simulink model "flightControlSystem"  (R2021a)
settings: Solver=ode3  StartTime=0  StopTime=TFinal  FixedStep=Ts  RelTol=1e-3  EnableMultiTasking=on
undefined symbols (not defined in the file): BINARIZATION_THRESHOLD, CHANGE_DERIVATIVE_ERROR_THRESHOLD_CURVE, CHANGE_DERIVATIVE_ERROR_THRESHOLD_STRAIGHT, codertarget, COG_X, COG_Y, Controller, DELAY_LANDING, DERIVATIVE_GAIN, DILATE_KERNEL, DiscIntNeverNeededParam, Discrete, DISK_KERNEL, Estimator, FLAG_WAIT_FOR_HOVERING, FOV, FRAME_SIZE_HEIGHT, FRAME_SIZE_WIDTH, g, G_B_GAIN, GAIN_LANDING, GAIN_TRACK, init, MAX_RADIUS_CROWN, MIN_RADIUS_CROWN, Sensors, strel, Time, TIME_HOLD, Ts, var_acc_angle_N, var_bias_gyr_N, var_gyro_p_N, Vehicle, Z_HIGH, Z_LOW
libraries: simulink x40, pid_lib x4, ctrlSharedLib x4, sharedtransform x3, visionmorphops x2, parrotlib x1
(part 3 of 3)

== matlab function flightControlSystem/Control System/Path Planning/MATLAB Function ==
  data: x_err_tr input; x_error output; y_err_tr input; x_err_ea input; y_err_ea input; flag_ho input; y_error output; flag_tl input
function [x_error, y_error] = decision_making(x_err_tr, y_err_tr, x_err_ea, ...
    y_err_ea, flag_ho, flag_tl)
% The MALTAB function sends the error along x- and y-axis to the non-linear 
% path planner. When the "flag_tl" is low, the position errors are computed
% as the difference between the end-marker and the drone CoG. Instead, when 
% the flag is high, the errors are computed by the difference between the 
% track and drone CoG.
%
% Inputs:
% - x_err_tr: tracking error along the x-axis. The error is expressed in 
% pixels.
% - y_err_tr: tracking error along the y-axis. The error is expressed in 
% pixels.
% - x_err_ea: position error along the x-axis when the end-marker is 
% detected. The error is expressed in pixels.
% - y_err_ea: position error along the y-axis when the end-marker is
% detected. The error is expressed in pixels.
% - flag_ho: the flag allows to check if the drone is able to fly.
% - flag_tl: the flag allows to trace the lane. 
%   
% Outputs
% - x_error: error between the drone CoG and the track/end-marker along the 
% x-axis. The error is expressed in pixels.
% - y_error: error between the drone CoG and the track/end-marker along the
% y-axis. The error is expressed in pixels

if flag_ho == 1
    
    if flag_tl == 0
        
        x_error = x_err_ea;
        y_error = y_err_ea;
        
    else
        
        x_error = x_err_tr;
        y_error = y_err_tr;

    end
    
else
    x_error = 0;
    y_error = 0;
    
end
    
end

== matlab function flightControlSystem/Image Processing System/track_VTP_generator ==
  data: frame input; error_y_track output; x_ref_prev input; y_ref_prev input; flag_track_prev input; error_x_track output; orientation_track output; flag_track output boolean; MIN_RADIUS_CROWN parameter; MAX_RADIUS_CROWN parameter; FOV parameter; COG_X parameter; COG_Y parameter
function [error_y_track, error_x_track, orientation_track, flag_track] = ...
track_VTP_generator(frame, x_ref_prev, y_ref_prev, flag_track_prev, ...
MIN_RADIUS_CROWN, MAX_RADIUS_CROWN, FOV, COG_X, COG_Y)
% The MATLAB function computes the error along x and y-axis between
% the drone COG (Center of Gravity) and the point of the track extract 
% by using of a crown circular mask. This errors is later used by the Path 
% Planner for the track tracking.  
%
%
% Inputs:
% - frame: binarized frame
% - x_ref_prev: previous value of the tracking point along the x-axis of 
% the track line. It is used as a reference for tracking the path.
% - y_ref_prev: previous value of the tracking point along the y-axis of 
% the track line. It is used as a reference for tracking the path.                                                                                                                                              
% - flag_track_prev: previous value assumed by the flag variablle, i.e., 
% the previous state of the drone (over the track / not over the track).
%
%
% Outputs:
% - error_y_track: error between the CoG of the drone and a point of the 
% lane in the forward direction along the y-axis. It is expressed in
% pixels.
% - error_x_track: error between the CoG of the drone and a point of the 
% lane in the forward direction along the x-axis. It is expressed in pixels. 
% - flag_track: it indicates if the drone is currently over the track (TRUE).
% - yaw: the heading angle of the track in the image plane.
%
%
% Parameters:
% - MIN_RADIUS_CROWN: minimum value of the radius of the crown mask. It is
% expressed in pixels.
% - MAX_RADIUS_CROWN: maximum value of the radius of the crown mask. It is
% expressed in pixels.
% - FOV: a portion of the crown used to detect the lane. It is expressed in
% radians.
% - COG_X: position of the drone CoG along x-axis of the reference frame.
% - COG_Y: position of the drone CoG along y-axis of the reference frame.

persistent x_accumulator
persistent y_accumulator
persistent pixel_count

if isempty(x_accumulator)
    x_accumulator = 0;
end

if isempty(y_accumulator)
    y_accumulator = 0;
end

if isempty(pixel_count)
    pixel_count = 0;
end

% the previous value of the heading angle of the lane 
orientation_track = atan2(-x_ref_prev,y_ref_prev); 
orientation_track = mod(orientation_track,2*pi);

% checking if the drone is over the lane
if flag_track_prev     

    % the set of pixels inside the crown mask
    for i = (COG_X-MAX_RADIUS_CROWN):(COG_X+MAX_RADIUS_CROWN) 

        for j = (COG_Y-MAX_RADIUS_CROWN):(COG_Y+MAX_RADIUS_CROWN)

            norm = sqrt(((i-(COG_X-0.5))^2)+((j-(COG_Y-0.5))^2));

            if norm >= MIN_RADIUS_CROWN && norm <= MAX_RADIUS_CROWN 

                axis_x = (i-(COG_X-0.5));
                axis_y = (j-(COG_Y-0.5));
                yaw_point_temp = atan2(axis_x,axis_y);


                yaw_point_temp_2 = mod(yaw_point_temp,2*pi);

                % a portion of the crown mask depending on the FOV
                threshold_1 = mod((orientation_track+(pi/FOV)),2*pi);

                threshold_2 = mod((orientation_track-(pi/FOV)),2*pi);

                if threshold_1 < threshold_2

                    flag_threshold = ...
                        (yaw_point_temp_2 <= 2*pi  && yaw_point_temp_2 >= threshold_2) ...
                        || (yaw_point_temp_2 <= threshold_1  && yaw_point_temp_2 >= 0);

                else

                    flag_threshold = ...
                        yaw_point_temp_2 <= threshold_1  && yaw_point_temp_2 >= threshold_2;

                end

                if flag_threshold
 
                    if frame(i,j)==1 
                        
                        pixel_count = pixel_count + 1;
                        x_accumulator = x_accumulator + i;
                        y_accumulator = y_accumulator + j;

                    end

                end

            end

        end
    end
    
else
    % checking for the initial heading angle of the lane. It can be 
    % different from the heading angle of the drone
    for i = (COG_X-MAX_RADIUS_CROWN):(COG_X+MAX_RADIUS_CROWN)

        for j = (COG_Y-MAX_RADIUS_CROWN):(COG_Y+MAX_RADIUS_CROWN)
            
            norm=sqrt(((i-(COG_X-0.5))^2)+((j-(COG_Y-0.5))^2));

            if norm>=MIN_RADIUS_CROWN && norm <= MAX_RADIUS_CROWN 

                 axis_x = (i-(COG_X-0.5));
                 axis_y = (j-(COG_Y-0.5));
                if frame(i,j)==1 
                    pixel_count=pixel_count +1;
                    x_accumulator=x_accumulator+i;
                    y_accumulator=y_accumulator+j;
                end
            end
        end
    end
end

% calculating the medium point of the lane as output of the mask
x_ref_temp = -(round(x_accumulator/pixel_count)-COG_X);
y_ref_temp = (round(y_accumulator/pixel_count)-COG_Y);

% when there is no track, the x_ref_temp and y_ref_temp variables are NaN.
% Below is the code for fix the issue.

if isnan(x_ref_temp)
    
    % if the computer vision algorithm does not detect the track, the 
    % drone position does not change
    error_x_track = 0 ;
    flag_error_x = false;
    
else
    
    % if the computer vision algorithm detects the track, a new position 
    % is computed for the tracking problem
    flag_error_x = true;
    error_x_track = x_ref_temp;
    
end

% As for the x coordinate
if isnan(y_ref_temp)
    
    error_y_track = 0 ;
    flag_error_y = false;
    
else
    
    error_y_track = y_ref_temp;
    flag_error_y=true ;
    
end

% checking if the drone is over the lane
flag_track = flag_error_x || flag_error_y;

% reset of the persistent variables
pixel_count = 0;
x_accumulator = 0;
y_accumulator = 0;

end

== stateflow chart flightControlSystem/Control System/Path Planning/circle count ==
  state State [group]
    - TAKE_OFF: The drone takes off and hovers.
    - LEAVE_MARKER: The drone leaves the marker through tracing the VTP set at the track.
    - TRACE_LANE: The drone traces either straight or curve line.
    - APPROACH_MARKER_CENTER: When the error between the drone CoG and the marker
    center is less than MAX_ERROR_LANDING, the drone flies down and then rises back.
  state INPUT [group]
    - flag_hover: flag raised when the drone is hovering within the altitude threshold.
    - flag_marker: flag raised when the marker is detected by the IPS.
  state OUTPUT [group]
    - cirlce_count: counting the circles that the drone has passed.
    - flag_tracelane: flag raised when the drone is going to track the lane.
  state TAKE_OFF
  state LEAVE_MARKER
    entry:
    flag_tracelane = 1;
  state TRACE_LANE
    entry:
    flag_tracelane = 1;
  state APPROACH_MARKER_CENTER
    entry:
    circle_count = circle_count +1
    flag_tracelane = 0
  (default) -> TAKE_OFF : {circle_count = 0, flag_tracelane = 0}
  TAKE_OFF -> LEAVE_MARKER : [after(3,sec) && flag_hover ==1]
  LEAVE_MARKER -> TRACE_LANE : [flag_hover == 1 && flag_end_marker == 0]
  APPROACH_MARKER_CENTER -> LEAVE_MARKER : [flag_hover == 0]
  TRACE_LANE -> APPROACH_MARKER_CENTER : [flag_end_marker == 1 ]
  data: flag_hover input; circle_count output; flag_end_marker input; flag_tracelane output

== matlab function flightControlSystem/Control System/Controller/Position Controller/Position error transformation (Earth to Body frame) ==
  data: yaw input; xy_err_earth input; xy_err_body output
function xy_err_body = fcn(yaw,xy_err_earth)

transformation = [cos(yaw), sin(yaw); -sin(yaw),  cos(yaw)];
xy_err_body = transformation * xy_err_earth;


end

== matlab function flightControlSystem/Control System/Path Planning/Non linear Path Planner/X_PLANNER/x_derivative_contribute /MATLAB Function ==
  data: derivative_error input; flag_change_error output; CHANGE_DERIVATIVE_ERROR_THRESHOLD input
function flag_change_error = change_error_checker(derivative_error, ...
    CHANGE_DERIVATIVE_ERROR_THRESHOLD)
% This MATLAB function recognizes if the derivative of the error is greater
% than a threshold value, i.e., the  CHANGE_DERIVATIVE_ERROR_THRESHOLD. 
% 
% Input:
% - derivative_error: derivative of the error. The error is expressed in 
% pixels
%
% Parameter:
% - CHANGE_DERIVATIVE_ERROR_THRESHOLD: threshold value.
%
% Output:
% - flag_change_error: flag raised when the derivative of the error
% changes.

if abs(derivative_error) >= CHANGE_DERIVATIVE_ERROR_THRESHOLD

    flag_change_error = 1;

else

    flag_change_error = 0;

end

== matlab function flightControlSystem/Control System/Path Planning/Non linear Path Planner/X_PLANNER/x_derivative_contribute /derivative error ==
  data: dev_contribute_prev input; derivative_error input; flag_change_error input; dev_contribute output; count_prev input; count output; flag_count_prev input; flag_count output; Ts parameter; TIME_HOLD parameter; DERIVATIVE_GAIN parameter
  function [dev_contribute, count, flag_count] = derivative_error(dev_contribute_prev, ...
    derivative_error, flag_change_error,count_prev,flag_count_prev, Ts, ...
    TIME_HOLD, DERIVATIVE_GAIN)
% This MATLAB function computes the derivative contribution of the path planner
% for the x coordinate.
%
% Inputs:
% - dev_contribute_prev: previous value derative part of the planner
% - derivative_error: derivative error value.
% - flag_change_error: it is raised when the sign of the error changes
% - count_prev: previous value of the counter. 
%
% Parameters:
% - Ts: sampling Time.
% - TIME_HOLD: time to which the previous value assumed by the derivative
% contribute has to be hold.
% - DERIVATIVE_GAIN: gain used for the derivative contribution.
%
% Output:
% - dev_contribute: derivative contribution of the path planner.
% - count: counter value
% - flag_count: flag raises when the derivate contribute does not more take
% part to the pat planner.

persistent count_to_be_hold

if isempty(count_to_be_hold)
    count_to_be_hold = round(TIME_HOLD/Ts);
end

flag_count = 0;

if flag_change_error && count_prev == 0    
    flag_count=1;   
end
   
if flag_count_prev || flag_count
    
    if count_prev == count_to_be_hold

        count=0;
        flag_count=0;

    else

        count=count_prev+1;
        flag_count=1;
        
    end
    
    dev_contribute=derivative_error*DERIVATIVE_GAIN;
    
    if dev_contribute ==0 && dev_contribute_prev ~=0 
        
        dev_contribute=dev_contribute_prev;
        
    end

else
    
    flag_count = 0;
    count = 0;
    dev_contribute = 0;
    
end

== stateflow chart flightControlSystem/Control System/Path Planning/Non linear Path Planner/X_PLANNER/x_linear_contribute ==
  state STATE [group]
    - TRACK_DETECTED: The Image Processing System detected the lane.
    - END_MARKER_DETECTED: The Image Processing System detected the end-marker.
  state INPUT [group]
    - Flag_track: flag raised when the lane is detected by the Image Processing System.
    - Flag_end_marker : flag raised when the end-marker is detected by the Image Processing System.
  state PARAMETERS [group]
    - GAIN_TRACK: gain used from the drone reference generator when it follows the lane.
    - GAIN_LANDING: gain used from the  drone reference generator for landing on the end-marker.
  state OUTPUT [group]
    - linear_part : linear contribute.
  state END_MARKER_DETECTED
    during:
    linear_part = error * GAIN_LANDING;
  state IDLE
  state TRACK_DETECTED
    during:
    linear_part = error * GAIN_TRACK;
  IDLE -> TRACK_DETECTED
  TRACK_DETECTED -> END_MARKER_DETECTED : [flag_end_marker==1 && flag_track==0]
  (default) -> IDLE
  data: error input double; GAIN_TRACK parameter double; GAIN_LANDING parameter double; flag_end_marker input double; flag_track input double; linear_part output double

== stateflow chart flightControlSystem/Control System/Path Planning/Non linear Path Planner/Y_PLANNER/Chart1 ==
  state STATE [group]
    - TAKE_OFF: The drone takes off and hovers.
    - LEAVE_MARKER: The drone leaves the marker through the VTP set at the track.
    - LINE_FOLLOWING: The drone follows either straight or curve line.
    - APPOACH_MARKER_CENTER: The drone approaches the circle center if the marker is deteced by the IPS.
    - PICK_EGG: When the error between the drone CoG and the marker center is less than MAX_ERROR_LANDING,
    the drone flies down and rises back.
  state INPUT [group]
    - flag_end_marker_to_Controller: flag raised when the drone has to land.
    - lin_part: linear part of the path planner.
    - dev_part: derivative part of the path planner.
    - y_estimated: estimated drone position along the y-axis.
    - flag_end_marker : flag raised when the marker is detected by the Image Processing System.
  state OUTPUT [group]
    - y_planned: y coordinate of the goal position.
  state LINE_FOLLOWING
    during:
    y_planned= y_estimated + lin_part + dev_part;
    y_planned_stored=y_planned;
  state LEAVE_MARKER
    during:
    y_planned= y_estimated + lin_part + dev_part;
    y_planned_stored=y_planned;
  state TAKE_OFF
    y_planned = 0;
  state PICK_EGG
    entry:
    y_planned=y_planned_stored;
  state APPROACH_MARKER_CENTER
    entry:
    circle_count = circle_count +1;
    during:
    y_planned= y_estimated + lin_part ;
    y_planned_stored=y_planned;
  (default) -> TAKE_OFF : {circle_count = 0, y_planned_stored = 0}
  TAKE_OFF -> LEAVE_MARKER : [after(3, sec) && flag_hover == 1]
  LEAVE_MARKER -> LINE_FOLLOWING : [flag_end_marker == 0]
  PICK_EGG -> LEAVE_MARKER : [after(5,sec) && flag_hover == 1 && circle_count <= 1]
  LINE_FOLLOWING -> APPROACH_MARKER_CENTER : [flag_end_marker == 1]
  APPROACH_MARKER_CENTER -> PICK_EGG : [flag_end_marker_to_controller==1]
  data: dev_part input double; lin_part input double; flag_end_marker_to_controller input double; flag_track input double; flag_end_marker input double; y_estimated input; y_planned_stored local double; y_planned output double; circle_count local double; flag_hover input

== matlab function flightControlSystem/Control System/Path Planning/Non linear Path Planner/Y_PLANNER/y_derivative_contribute /MATLAB Function ==
  data: derivative_error input; flag_change_error output; CHANGE_DERIVATIVE_ERROR_THRESHOLD input
function flag_change_error = change_error_checker(derivative_error, ...
    CHANGE_DERIVATIVE_ERROR_THRESHOLD)
% This MATLAB function recognizes if the derivative of the error is greater
% than a threshold value, i.e., the  CHANGE_DERIVATIVE_ERROR_THRESHOLD. 
% 
% Input:
% - derivative_error: derivative of the error. The error is expressed in 
% pixels
%
% Parameter:
% - CHANGE_DERIVATIVE_ERROR_THRESHOLD: threshold value.
%
% Output:
% - flag_change_error: flag raised when the derivative of the error
% changes.

if abs(derivative_error) >= CHANGE_DERIVATIVE_ERROR_THRESHOLD

    flag_change_error = 1;

else

    flag_change_error = 0;

end

== matlab function flightControlSystem/Control System/Path Planning/Non linear Path Planner/Y_PLANNER/y_derivative_contribute /derivative error ==
  data: dev_contribute_prev input; derivative_error input; flag_change_error input; dev_contribute output; count_prev input; count output; flag_count_prev input; flag_count output; Ts parameter; TIME_HOLD parameter; DERIVATIVE_GAIN parameter
function [dev_contribute, count, flag_count] = derivative_error(dev_contribute_prev, ...
    derivative_error, flag_change_error,count_prev,flag_count_prev, Ts, ...
    TIME_HOLD, DERIVATIVE_GAIN)
% This MATLAB function computes the derivative contribution of the path planner
% for the x coordinate.
%
% Inputs:
% - dev_contribute_prev: previous value derative part of the planner
% - derivative_error: derivative error value.
% - flag_change_error: it is raised when the sign of the error changes
% - count_prev: previous value of the counter. 
%
% Parameters:
% - Ts: sampling Time.
% - TIME_HOLD: time to which the previous value assumed by the derivative
% contribute has to be hold.
% - DERIVATIVE_GAIN: gain used for the derivative contribution.
%
% Output:
% - dev_contribute: derivative contribution of the path planner.
% - count: counter value
% - flag_count: flag raises when the derivate contribute does not more take
% part to the pat planner.

persistent count_to_be_hold

if isempty(count_to_be_hold)
    count_to_be_hold = round(TIME_HOLD/Ts);
end

flag_count = 0;

if flag_change_error && count_prev == 0    
    flag_count=1;   
end
   
if flag_count_prev || flag_count
    
    if count_prev == count_to_be_hold

        count=0;
        flag_count=0;

    else

        count=count_prev+1;
        flag_count=1;
        
    end
    
    dev_contribute=derivative_error*DERIVATIVE_GAIN;
    
    if dev_contribute ==0 && dev_contribute_prev ~=0 
        
        dev_contribute=dev_contribute_prev;
        
    end

else
    
    flag_count = 0;
    count = 0;
    dev_contribute = 0;
    
end

== stateflow chart flightControlSystem/Control System/Path Planning/Non linear Path Planner/Y_PLANNER/y_linear_contribute ==
  state STATE [group]
    - TRACKING: the drone is tracking the lane or the marker.
    - LANDING: the drone lands when the marker is detected and the error between the drone CoG and the marker center
    is less than MAX_ERROR_LANDING.
    - TRACK_DETECTED: the Image Processing System detects the lane.
    - END_MARKER_DETECTED: the Image Processing System detects the marker.
  state INPUT [group]
    - flag_track: flag raised when the lane is detected by Image Processing System.
    - flag_end_marker_to_controller: flag raised when the drone has to land.
    - lin_part: linear part of the path planner.
    - dev_part: derivative part of the path planner.
    - y_estimated: y coordinate of the drone position.
    - flag_end_marker: flag raised when the marker is detected by Image Processing System.
  state PARAMETERS [group]
    - GAIN_TRACK: gain used by the drone reference generator to follow the lane.
    - GAIN_LANDING: gain used by the drone reference generator to land over the marker.
  state OUTPUT [group]
    - y_planned: y coordinate of the goal position.
  state END_MARKER_DETECTED
    during:
    linear_part = error * GAIN_LANDING;
  state IDLE
  state TRACK_DETECTED
    during:
    linear_part = error * GAIN_TRACK;
  TRACK_DETECTED -> END_MARKER_DETECTED : [flag_end_marker==1 && flag_track==0]
  IDLE -> TRACK_DETECTED : [flag_end_marker==1 && flag_track==0]
  (default) -> IDLE
  data: error input double; GAIN_TRACK parameter double; GAIN_LANDING parameter double; flag_end_marker input double; flag_track input double; linear_part output double

== stateflow chart flightControlSystem/Control System/Path Planning/Non linear Path Planner/Z PLANNER/Chart ==
  state STATE [group]
    - TAKE-OFF： The drone takes off and hovers at 0.7m.
    - TRACKING: The drone is tracking the lane or the marker when they are detected.
    - PICK_EGG: When the error between the drone CoG and the marker center is less than the MAX_ERROR_LANDING,
    the drone flies down.
    - LANDING: The drons lands when the final marker is detected.
  state INPUT [group]
    - flag_end_marker: flag raised when the end-marker is detected by the Image Processing System.
    - norm error: error between the drone CoG and the central point of the end-marker.
  state OUTPUT [group]
    - z_planned: drone altitude sent to the drone controller.
    - flag_end_marker_to_controller: flag raise when the drone has to land.
  state PICK_EGG
    entry:
    z_planned =  -0.5;
    flag_end_marker_to_controller=1;
    circle_count = circle_count +1;
  state LANDING
    entry:
    z_planned = 0;
  state TRACKING
    entry:
    z_planned =  -0.7  ;
    flag_end_marker_to_controller=0;
  state TAKE_OFF
    entry:
    z_planned =  -0.7 ;
    flag_end_marker_to_controller = 0;
  (default) -> TAKE_OFF : {circle_count = 0}
  PICK_EGG -> LANDING [order 2] : [circle_count >1]
  TRACKING -> PICK_EGG : [flag_end_marker==1 && norm_error <= MAX_ERROR_LANDING]
  TAKE_OFF -> TRACKING : [after(3,sec) && flag_hover == 1&& flag_end_marker == 0]
  PICK_EGG -> TAKE_OFF [order 1] : [after(3,sec)&& circle_count <=1]
  data: norm_error input double; z_planned output double; MAX_ERROR_LANDING parameter double; flag_end_marker input; flag_end_marker_to_controller output double; flag_hover input; circle_count local double

== matlab function flightControlSystem/Control System/Path Planning/Non linear Path Planner/Z PLANNER/MATLAB Function ==
  data: norm_error_tot output; error_x input; norm_error output; error_y input; flag_end_marker input; norm_error_prev input
function [norm_error_tot, norm_error] = error_function(error_x, error_y, ...
flag_end_marker, norm_error_prev)
% This MATLAB function computes the norm of the error between the drone CoG
% drone and the middle of point of the end-marker. The norm error is
% computed only if the end-marker is detected.
%
%
%Inputs:
% - error_x: error along the x-axis between the drone CoG and the central 
% point of the end-marker.
% - error_y: error along the y-axis between the drone CoG and the central 
% point of the end-marker.
% - flag_end_marker: the flag indicates when the end-marker is detected.
% - norm_error_prev: previous value of the norm of the error.                                                                                                                                              
%  
%
%Outputs:
% - norm_error_tot: norm of the error between the drone CoG and the central 
% point of the end-marker. It consideres the previous value assumed by the
% norm of the error. The values is condisdered  at the time k = time_step +
% DELAY_LANDING \cdot sampling time. 
% - norm_error: actual value assumed by the norm of error. The error is 
% computed by the drone CoG and the middle point of the end-marker.

if flag_end_marker
    
    norm_error = sqrt((error_x)^2 + (error_y)^2);
    norm_error_tot = norm_error + norm_error_prev  ;
    
else 
    %100 is a constant value greater than MAX_ERROR_LANDING
    norm_error_tot = 100;
    norm_error = 100;
end

== matlab function flightControlSystem/Image Processing System/Image Binarization ==
  data: r input; binarized_frame output; g input; b input; G_B_GAIN parameter; BINARIZATION_THRESHOLD parameter
function binarized_frame = binarizer(r, g, b,G_B_GAIN, BINARIZATION_THRESHOLD)
% The MATLAB function computes a binarized frame starting from a frame 
% expressed in the RGB file format. 
%
% Inputs:
% - r: Red channel frame
% - g: Green channel frame
% - b: Blue channel frame
%
% Output:
% - binarze_frame: the binarized frame
%
% Parameters:
% - G_B_GAIN: used to reduce the amount of green and blue colors inside the frame
% - BINARIZER_THRESHOLD: threshold to detect only the track inside the frame 

frame= r - (g/G_B_GAIN) - (b/G_B_GAIN);

binarized_frame = frame >= BINARIZATION_THRESHOLD;

end

== matlab function flightControlSystem/Image Processing System/MATLAB Function ==
  data: marker_frame input; binarized_frame input; frame output
function frame = trackerosion(marker_frame, binarized_frame)
% The MATLAB function computes the track frame.
%
% Input:
% - marker_frame: the seperated marker frame obtained as the convolution 
% with a disk kernel
%
% Output:
% - binarized_frame: the binarized image frame, including both of marker 
% and track 

frame = binarized_frame - marker_frame;
end

== matlab function flightControlSystem/Image Processing System/Red Marker VTP generator ==
  data: center_x output; center_y output; binary input; error_x_end_marker output; FRAME_SIZE_WIDTH parameter; FRAME_SIZE_HEIGHT parameter; COG_X parameter; COG_Y parameter; error_y_end_marker output; flag_marker output
function [center_x,center_y,error_x_end_marker, error_y_end_marker, flag_marker]...
    = red_marker_VTP_generator(binary,FRAME_SIZE_WIDTH,... 
FRAME_SIZE_HEIGHT,COG_X, COG_Y)
% The MATLAB function computes the errors along the x- and y-axis between
% the drone COG(Center of Gravity and the middle of the lane. The red marker is detected by 
% using a disk kernel. 
%
%
% Inputs:
% - binary: binarized frame obtained as the convolution with a disk kernel
%
% Outputs:
% - center_x: the x-axis of the detected marker's center.
% - center_y: the y-axis of the detected marker's center.
% - error_y_end_marker: error between the CoG of the drone and a point of the 
% lane in the forward direction along the y-axis. It is expressed in
% pixels.
% - error_x_end_maker: error between the CoG of the drone and a point of the 
% lane in the forward direction along the x-axis. It is expressed in pixels. 
% - flag_marker: it is TURE if the Image Processing System detects 
% the marker.
% 
%
%
%Parameters:
% - COG_X: position of the drone CoG along x-axis of the reference frame.
% - COG_Y: position of the drone CoG along y-axis of the reference frame.
% - FRAME_SIZE_WIDTH: width of the frame.
% - FRAME_SIZE_HEIGHT: height of the frame.

persistent column_accumulator
persistent count_pixel
persistent row_accumulator




if isempty(column_accumulator)
    column_accumulator = 0;
end

if isempty(count_pixel)
    count_pixel = 0;
end

if isempty(row_accumulator)
    row_accumulator = 0;
end

%accumulate all the circle pixels
for i=1:FRAME_SIZE_HEIGHT

    for j=1:FRAME_SIZE_WIDTH

        %check all the pixel belonging to the end marker
        if binary(i,j)==1
            count_pixel = count_pixel +1;
            column_accumulator = column_accumulator + j;
            row_accumulator = row_accumulator + i;

        end

    end
end

%check if a marker is detected
if count_pixel ~=0
    flag_marker = 1;
    center_x = round(row_accumulator/count_pixel)-5;
    center_y = round(column_accumulator/count_pixel);
else
    flag_marker=0;
    center_x = COG_X;
    center_y = COG_Y;
end


% Calculate the medium point of the end marker
error_x_end_marker = -(center_x - COG_X);
error_y_end_marker = (center_y - COG_Y);





% reset of the persistent variables
column_accumulator = 0;
row_accumulator = 0;
count_pixel = 0;


end
